simulink model "velauto"  (Simulink 8.1)
settings: Solver=ode45  StartTime=0.0  StopTime=150  RelTol=1e-3
libraries: fuzblock x1
settings Model: Creator=BLUE  LastModifiedBy=BLUE
settings DataIOCC: SignalLoggingSaveFormat=Dataset
settings OptimizationCC: ExpressionDepthLimit=128
settings DebuggingCC: FcnCallInpInsideContextMsg=EnableAllAsError
settings GRTTargetCC: CombineOutputUpdateFcns=on  GRTInterface=off

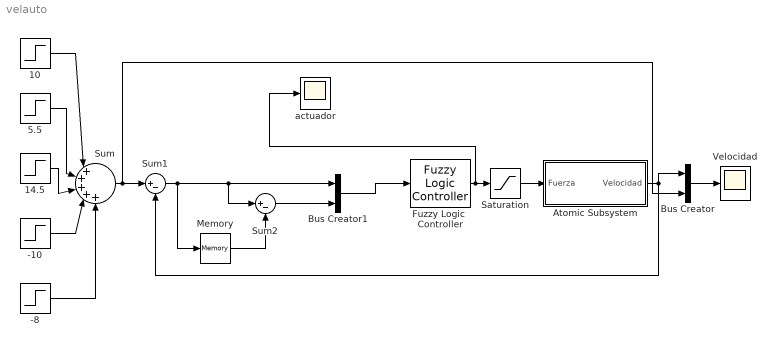
== system velauto ==
  "-10    " : Step  Time=90  After=-10  SampleTime=0
  "-8   " : Step  Time=120  After=-8  SampleTime=0
  "10  " : Step  Time=0  After=10  SampleTime=0
  "14.5   " : Step  Time=30  After=14.5  SampleTime=0
  "5.5   " : Step  Time=15  After=5.5  SampleTime=0
  Atomic Subsystem : Subsystem
      settings: RTWSystemCode=Nonreusable function
  Bus Creator : BusCreator  Inputs=2
  Bus Creator1 : BusCreator  Inputs=2
  Fuzzy Logic  Controller : fuzblock/Fuzzy Logic  Controller  fis=[]
  Memory : Memory
  Saturation : Saturate  UpperLimit=1600  LowerLimit=0
  Sum : Sum  Inputs=|+++++
  Sum1 : Sum  Inputs=|+-
  Sum2 : Sum  Inputs=|+-
  "Velocidad " : Scope
      settings: YMin=2.5  YMax=10.5
  "actuador " : Scope
      settings: TimeRange=150  YMin=0  YMax=40
  wires:
  Fuzzy Logic  Controller/1 -> "actuador "/1, Saturation/1
  Saturation/1 -> Atomic Subsystem/1(Fuerza)
  "10  "/1 -> Sum/1
  "5.5   "/1 -> Sum/2
  "14.5   "/1 -> Sum/3
  "-10    "/1 -> Sum/4
  "-8   "/1 -> Sum/5
  Sum/1 -> Bus Creator/2, Sum1/1
  Bus Creator/1 -> "Velocidad "/1
  Sum1/1 -> Memory/1, Sum2/1, Bus Creator1/1
  Memory/1 -> Sum2/2
  Atomic Subsystem/1("Velocidad ") -> Sum1/2, Bus Creator/1
  Sum2/1 -> Bus Creator1/2
  Bus Creator1/1 -> Fuzzy Logic  Controller/1

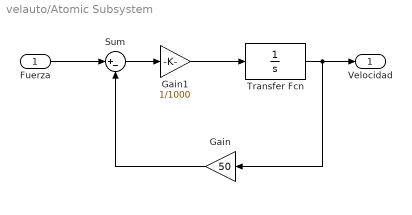
== system velauto/Atomic Subsystem ==
  Fuerza : Inport
  Gain : Gain  Gain=50
  Gain1 : Gain  Gain=1/1000
  Sum : Sum  Inputs=|+-
  Transfer Fcn : TransferFcn  Denominator=[1 0]
  "Velocidad " : Outport
  wires:
  Gain/1 -> Sum/2
  Fuerza/1 -> Sum/1
  Sum/1 -> Gain1/1
  Gain1/1 -> Transfer Fcn/1
  Transfer Fcn/1 -> Gain/1, "Velocidad "/1
